simulink model "ASV_pathplot"  (Simulink 7.7)
settings: Solver=FixedStepDiscrete  SolverMode=SingleTasking  StartTime=0.0  StopTime=100  FixedStep=sampletime  RelTol=1e-3
model workspace (MAT data in the model file):
  sampletime : num (value not decoded)
PostLoadFcn:
  | open('ASV_pathplot_GUI.fig')
StartFcn:
  | listener = @OriCallback
  | 
  | rto_ori = add_exec_event_listener('ASV_pathplot/Orientation','PostOutputs',listener)
  | rto_speed = add_exec_event_listener('ASV_pathplot/Speed','PostOutputs',@SpeedCallback)
StopFcn:
  | clear rto*
undefined symbols (not defined in the file or in its folder): DiscIntNeverNeededParam, magnitude
libraries: simulink x2, SimulinkExecutionControl x1
settings Model: Creator=Fodi  LastModifiedBy=Fodi

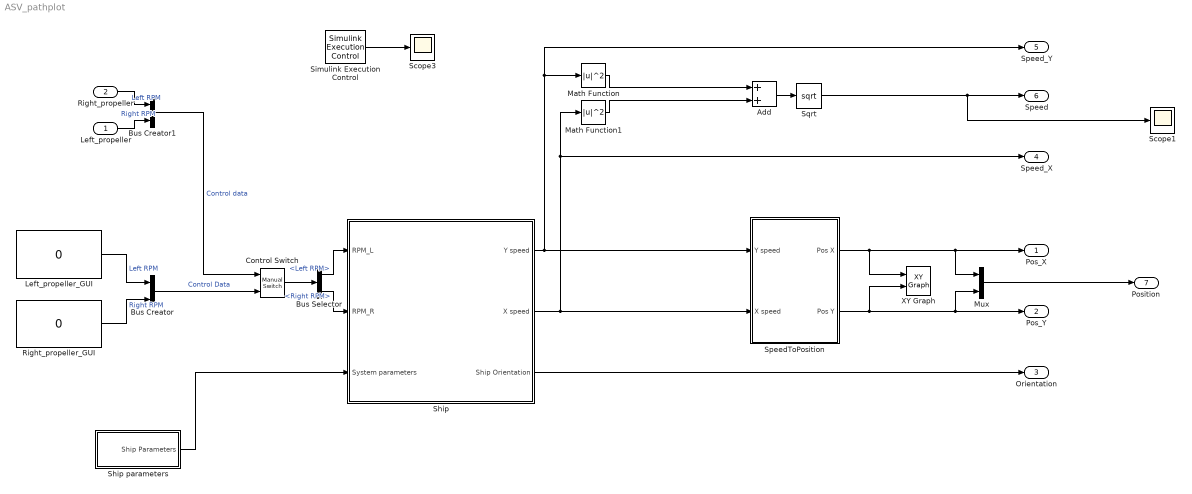
== system ASV_pathplot ==
  Left_propeller : Inport
  Right_propeller : Inport  Port=2
  Add : Sum
  Bus Creator : BusCreator  Inputs=2
  Bus Creator1 : BusCreator  Inputs=2
  Bus Selector : BusSelector  OutputSignals=Left RPM,Right RPM
  Control Switch : simulink/Signal Routing/Manual Switch  SystemSampleTime=-1  sw=0  action=0  varsize=off
  Left_propeller_GUI : Constant  Value=0  OutDataTypeStr=double
  Math Function : Math  Operator=magnitude^2  SaturateOnIntegerOverflow=on
  Math Function1 : Math  Operator=magnitude^2  SaturateOnIntegerOverflow=on
  Mux : Mux  Inputs=2
  Right_propeller_GUI : Constant  Value=0  OutDataTypeStr=double
  Scope1 : Scope
  Scope3 : Scope
      settings: SaveName=ScopeData14
  Ship : Subsystem
  Ship parameters : Subsystem
  Simulink Execution Control : SimulinkExecutionControl/Simulink Execution Control  SystemSampleTime=-1  proc_pri=NORMAL_PRIORITY_CLASS  thread_pri=THREAD_PRIORITY_NORMAL  rt_sim=on  factor=1  ovrrun=Continue execution  Ts=sampletime
  SpeedToPosition : Subsystem
  Sqrt : Sqrt  SaturateOnIntegerOverflow=on
  XY Graph : simulink/Sinks/XY Graph  SystemSampleTime=-1  xmin=-100  xmax=100  ymin=-100  ymax=100  st=-1
  Pos_X : Outport
  Pos_Y : Outport  Port=2
  Orientation : Outport  Port=3
  Speed_X : Outport  Port=4
  Speed_Y : Outport  Port=5
  Speed : Outport  Port=6
  Position : Outport  Port=7
  wires:
  Ship parameters/1(Ship Parameters) -> Ship/3(System parameters)
  Ship/2(X speed) -> SpeedToPosition/2(X speed), Math Function1/1, Speed_X/1
  Ship/1(Y speed) -> SpeedToPosition/1(Y speed), Speed_Y/1, Math Function/1
  Simulink Execution Control/1 -> Scope3/1
  SpeedToPosition/1(Pos X) -> XY Graph/1, Pos_X/1, Mux/1
  SpeedToPosition/2(Pos Y) -> XY Graph/2, Pos_Y/1, Mux/2
  Left_propeller_GUI/1 -> Bus Creator/1  "Left RPM"
  Right_propeller_GUI/1 -> Bus Creator/2  "Right RPM"
  Right_propeller/1 -> Bus Creator1/1  "Left RPM"
  Left_propeller/1 -> Bus Creator1/2  "Right RPM"
  Bus Creator1/1 -> Control Switch/1  "Control data"
  Bus Creator/1 -> Control Switch/2  "Control Data"
  Control Switch/1 -> Bus Selector/1
  Bus Selector/1 -> Ship/1(RPM_L)  "<Left RPM>"
  Bus Selector/2 -> Ship/2(RPM_R)  "<Right RPM>"
  Add/1 -> Sqrt/1
  Sqrt/1 -> Speed/1, Scope1/1
  Math Function/1 -> Add/1
  Math Function1/1 -> Add/2
  Ship/3(Ship Orientation) -> Orientation/1
  Mux/1 -> Position/1

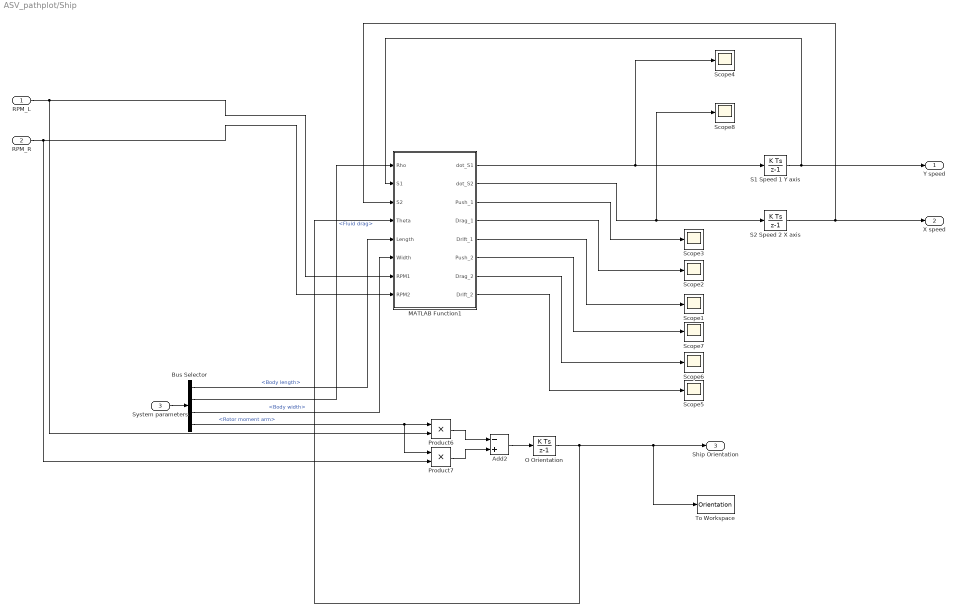
== system ASV_pathplot/Ship ==
  RPM_L : Inport
  RPM_R : Inport  Port=2
  System parameters : Inport  Port=3
  Add2 : Sum  Inputs=-+
  Bus Selector : BusSelector  OutputSignals=Ship Geometry.Body length,Water parameters.Fluid drag,Ship Geometry.Body width,Ship Geometry.Rotor moment arm
  MATLAB Function1 : Stateflow chart  TreatAsAtomicUnit=on
  O Orientation : DiscreteIntegrator  SampleTime=sampletime  ICPrevOutput=DiscIntNeverNeededParam  ICPrevScaledInput=DiscIntNeverNeededParam
  Product6 : Product  RndMeth=Zero
  Product7 : Product  RndMeth=Zero
  S1 Speed 1 Y axis : DiscreteIntegrator  SampleTime=sampletime  ICPrevOutput=DiscIntNeverNeededParam  ICPrevScaledInput=DiscIntNeverNeededParam
  S2 Speed 2 X axis : DiscreteIntegrator  InitialCondition=0.1  SampleTime=sampletime  ICPrevOutput=DiscIntNeverNeededParam  ICPrevScaledInput=DiscIntNeverNeededParam
  Scope{1..8} (8 alike) : Scope
      Scope1 settings: SaveName=ScopeData6
      Scope2 settings: SaveName=ScopeData7
      Scope3 settings: SaveName=ScopeData8
      Scope4 settings: SaveName=ScopeData9
      Scope5 settings: SaveName=ScopeData10
      Scope6 settings: SaveName=ScopeData11
      Scope7 settings: SaveName=ScopeData12
      Scope8 settings: SaveName=ScopeData13
  To Workspace : ToWorkspace  VariableName=Orientation  SampleTime=-1  SaveFormat=Structure
      settings: MaxDataPoints=1
  Y speed : Outport
  X speed : Outport  Port=2
  Ship Orientation : Outport  Port=3
  wires:
  S1 Speed 1 Y axis/1 -> Y speed/1, MATLAB Function1/2(S1)
  S2 Speed 2 X axis/1 -> X speed/1, MATLAB Function1/3(S2)
  RPM_L/1 -> Product6/2, MATLAB Function1/7(RPM1)
  RPM_R/1 -> Product7/2, MATLAB Function1/8(RPM2)
  O Orientation/1 -> MATLAB Function1/4(Theta), Ship Orientation/1, To Workspace/1
  System parameters/1 -> Bus Selector/1
  Add2/1 -> O Orientation/1
  Product6/1 -> Add2/1
  Product7/1 -> Add2/2
  Bus Selector/4 -> Product6/1, Product7/1  "<Rotor moment arm>"
  Bus Selector/1 -> MATLAB Function1/5(Length)  "<Body length>"
  Bus Selector/3 -> MATLAB Function1/6(Width)  "<Body width>"
  Bus Selector/2 -> MATLAB Function1/1(Rho)  "<Fluid drag>"
  MATLAB Function1/1(dot_S1) -> S1 Speed 1 Y axis/1, Scope4/1
  MATLAB Function1/2(dot_S2) -> S2 Speed 2 X axis/1, Scope8/1
  MATLAB Function1/3(Push_1) -> Scope3/1
  MATLAB Function1/4(Drag_1) -> Scope2/1
  MATLAB Function1/5(Drift_1) -> Scope1/1
  MATLAB Function1/6(Push_2) -> Scope7/1
  MATLAB Function1/7(Drag_2) -> Scope6/1
  MATLAB Function1/8(Drift_2) -> Scope5/1

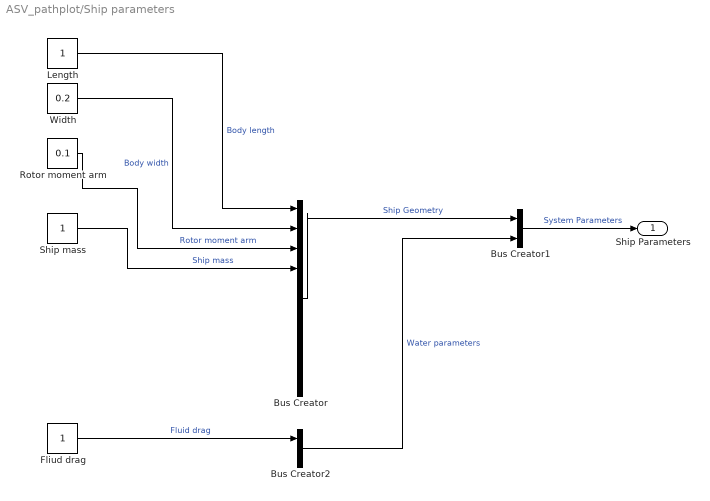
== system ASV_pathplot/Ship parameters ==
  Bus Creator : BusCreator  Inputs=10
  Bus Creator1 : BusCreator  Inputs=2
  Bus Creator2 : BusCreator  Inputs=2
  Fliud drag : Constant
  Length : Constant
  Rotor moment arm : Constant  Value=0.1
  Ship mass : Constant
  Width : Constant  Value=0.2
  Ship Parameters : Outport
  wires:
  Length/1 -> Bus Creator/1  "Body length"
  Width/1 -> Bus Creator/2  "Body width"
  Bus Creator/1 -> Bus Creator1/1  "Ship Geometry"
  Bus Creator1/1 -> Ship Parameters/1  "System Parameters"
  Bus Creator2/1 -> Bus Creator1/2  "Water parameters"
  Fliud drag/1 -> Bus Creator2/1  "Fluid drag"
  Rotor moment arm/1 -> Bus Creator/3  "Rotor moment arm"
  Ship mass/1 -> Bus Creator/4  "Ship mass"

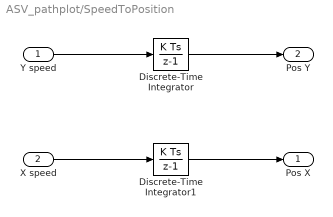
== system ASV_pathplot/SpeedToPosition ==
  Y speed : Inport
  X speed : Inport  Port=2
  Discrete-Time Integrator : DiscreteIntegrator  SampleTime=sampletime  ICPrevOutput=DiscIntNeverNeededParam  ICPrevScaledInput=DiscIntNeverNeededParam
  Discrete-Time Integrator1 : DiscreteIntegrator  SampleTime=sampletime  ICPrevOutput=DiscIntNeverNeededParam  ICPrevScaledInput=DiscIntNeverNeededParam
  Pos X : Outport
  Pos Y : Outport  Port=2
  wires:
  Y speed/1 -> Discrete-Time Integrator/1
  Discrete-Time Integrator/1 -> Pos Y/1
  X speed/1 -> Discrete-Time Integrator1/1
  Discrete-Time Integrator1/1 -> Pos X/1

== matlab function Ship/MATLAB Function1 ==
  data: Rho input double; dot_S1 output double; S1 input double; S2 input double; Theta input double; Length input double; Width input double; dot_S2 output double; Push_1 output double; RPM1 input double; RPM2 input double; Drag_1 output double; Drift_1 output double; Push_2 output double; Drag_2 output double; Drift_2 output double
function [dot_S1,dot_S2,Push_1,Drag_1,Drift_1,Push_2,Drag_2,Drift_2] = Dynamics(Rho, S1, S2, Theta, Length, Width, RPM1, RPM2)
%#codegen

Push_1 = (RPM1 + RPM2) * sin(Theta);
Drift_1 = (S1 * abs(cos(Theta)) - 0.1 * S2 * sin(Theta)) * Rho * Length;
Drag_1 = Rho * Width * S1 * abs(sin (Theta));

dot_S1 = Push_1 - Drag_1 - Drift_1;

Push_2 = (RPM1 + RPM2) * cos(Theta);
Drift_2 = (S2 * abs(sin(Theta)) - 0.1 * S1 * sin(Theta)) * Rho * Length;
Drag_2 = Rho * Width * S2 * abs(cos(Theta));

dot_S2 = Push_2 - Drag_2 - Drift_2;
